simulink model "Subsystem"  (R2020b)
settings: Solver=VariableStepAuto  StartTime=0.0  StopTime=10.0  RelTol=1e-3
settings Model: DataDictionary=W2_Prob4.sldd  Creator=kshir  LastModifiedBy=kshir
settings DataIOCC: SaveOutput=off  SaveTime=off

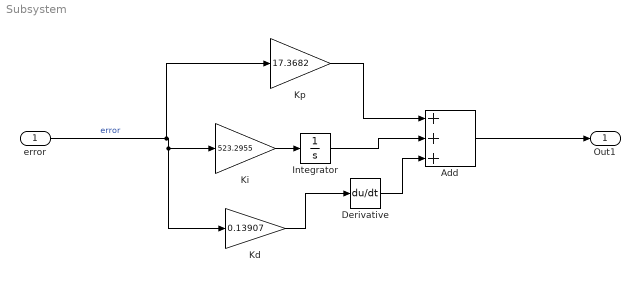
== system Subsystem ==
  error : Inport  OutDataTypeStr=double  PortDimensions=1  SampleTime=0
  Add : Sum  Inputs=+++
  Derivative : Derivative
  Integrator : Integrator
  Kd : Gain  Gain=0.13907
  Ki : Gain  Gain=523.2955
  Kp : Gain  Gain=17.3682
  Out1 : Outport  OutDataTypeStr=double  PortDimensions=1  SampleTime=0
  wires:
  Ki/1 -> Integrator/1
  Integrator/1 -> Add/2
  error/1 -> Kp/1, Ki/1, Kd/1  "error"
  Kd/1 -> Derivative/1
  Kp/1 -> Add/1
  Add/1 -> Out1/1
  Derivative/1 -> Add/3
